simulink model "PubIfDecisionTOS_MDL"  (R2020b)
settings: configuration reference "DspaceConfig" (kept outside this file)
PostLoadFcn:
  | if any(exist('dsrtsu_mdlpostloadfcn', 'file') ~= 0), dsrtsu_mdlpostloadfcn('Execute', bdroot); end
InitFcn:
  | , if any(exist('dsmpb_private', 'file') ~= 0), dsmpb_private('dsmpb_mdlclblib', 'Init', bdroot); end,
undefined symbols (not defined in the file or in its folder): C_TOS_ACCEgoRAxletoFbumplength_m, C_TOS_ACCTargetFront_Flag, C_TOS_AEBJAPedObjDxThre_Val, C_TOS_AEBJAPedObjDyThre_Val, C_TOS_AEBJATargetSize_Val, C_TOS_AEBJAVehObjDxThre_Val, C_TOS_AEBJAVehObjDyThre_Val, C_TOS_AEBJuncPedTargetSize_Val, C_TOS_AEBLatObjDxThre_Val, C_TOS_AEBLatPedDyThre_Val, C_TOS_AEBLatTargetSize_Val, C_TOS_AEBLongTargetInEgoFront_Flag, C_TOS_axAbsGround_Parameter, C_TOS_CameraConfirmedFlag, C_TOS_CNsubjWidth, C_TOS_CurrentLaneCoreMinWidth_Val, C_TOS_CutInProb_Val_Zero, C_TOS_CutOutProb_Val_Zero, C_TOS_D2R_Val, C_TOS_DefaultValueObjectToCenterLine_dy, C_TOS_EgoCarWidth_Val, C_TOS_EgoDxRefPoint_m, C_TOS_EgoRAxletoFbumplength_m, C_TOS_HalfWidthVehicle_Con, C_TOS_HWA_CurrentLaneFlag, C_TOS_HWA_LeftLaneFlag, C_TOS_HWA_MovingDir_Vaild, C_TOS_HWA_MovState_Vaild, C_TOS_HWA_RightLaneFlag, C_TOS_LaneLineCourseErrorFront, C_TOS_LaneLineCourseErrorRear, C_TOS_MotorbikeDefaultWidth_m, C_TOS_NumberOfEffectiveTargets, C_TOS_Obj_Age_Val, C_TOS_Objdx_Constraint_Val, C_TOS_ObjectDefaultWidth_m, C_TOS_ObjInCurrentLane_Val, C_TOS_ObjInCurrentLaneValid, C_TOS_ObjInLeftLaneValid, C_TOS_ObjInRightLaneValid, C_TOS_ObjNotInCurrentLane_Val, C_TOS_ObjNotREElementType, C_TOS_ObjPredictDis_dy_ConstantVal_Zeros, C_TOS_ObjToCenterLine_ConstantVal_Zeros, C_TOS_OFMObjIDInvilad_Val, C_TOS_PIL_LatDisCons_Val_zero, C_TOS_PIL_ObjectCutInFlag_b, C_TOS_PIL_ObjectCutOutFlag_b, C_TOS_PIL_ObjLaneProb_al_Val, C_TOS_PP_ObjFusType_FC_Confirm_b, C_TOS_PP_ObjFusType_FC_FR_Confirm_b, C_TOS_PP_ObjFusType_FR_Confirm_b, C_TOS_RE_80BoolDefault_Val, C_TOS_RE_80Single181Default_Val, C_TOS_RE_80Single255Default_Val, C_TOS_RE_80Uint8Default_Val, C_TOS_RE_D2R, C_TOS_RE_D_180_Val, C_TOS_RE_InvalidObjectID_Val, C_TOS_RE_InvalidTargetChainDir_Val ... (+142)
libraries: simulink x1650, TOS_LIB x361, canfdmsglib x14
(part 27 of 69)

== system PubIfDecisionTOS_MDL/TOS_20201112/TOS_2012080320/TOS/ACC/TOS_ACCCurrentLane/ACC_CurrentLane_Target/TOS_ACC_P0/ACC_P0_Targe ==
  ACC_P0_Index : Inport
  Object_Fus_Type : Inport  Port=2
  object_MovingState : Inport  Port=3
  PP_ObjMovingDirSignalProcessing : Inport  Port=4
  Object_HeadingAngle : Inport  Port=5
  Object_DX : Inport  Port=6
  TOS_TLJ_SameLaneConfirm_Flag : Inport  Port=7
  Object_Type : Inport  Port=8
  Object_ObstacleProb : Inport  Port=9
  Object_DY : Inport  Port=10
  PP_ObjFusType_FC_FR_Confirm : Inport  Port=11
  PP_ObjFusType_FR_Confirm : Inport  Port=12
  PP_ObjFusType_FC_Confirm : Inport  Port=13
  Object_VX : Inport  Port=14
  Object_VY : Inport  Port=15
  VIE_EgoVelocity : Inport  Port=16
  SteerWheelAng : Inport  Port=17
  PIL_OverlapRatio : Inport  Port=18
  ACC_Target_ID_K1 : Inport  Port=19
  ACC_Target_ID_K2 : Inport  Port=20
  ACC_Target_MovState_K1 : Inport  Port=21
  ACC_Target_MovState_K2 : Inport  Port=22
  ObjectID : Inport  Port=23
  LM_LR_Line04_dDisStart : Inport  Port=24
  LM_LR_Line04_dDisEnd : Inport  Port=25
  LM_LR_Line05_dDisStart : Inport  Port=26
  LM_LR_Line05_dDisEnd : Inport  Port=27
  LM_LR_Line06_dDisStart : Inport  Port=28
  LM_LR_Line06_dDisEnd : Inport  Port=29
  LM_LR_Line04_pC2 : Inport  Port=30
  LM_LR_Line05_pC2 : Inport  Port=31
  LM_LR_Line06_pC2 : Inport  Port=32
  LM_LR_Line04_fCamValid : Inport  Port=33
  LM_LR_Line05_fCamValid : Inport  Port=34
  LM_LR_Line06_fCamValid : Inport  Port=35
  LM_LR_Line04_pC0 : Inport  Port=36
  LM_RL_Line04_pC0 : Inport  Port=37
  LM_LR_Line04_pC1 : Inport  Port=38
  LM_RL_Line04_pC1 : Inport  Port=39
  Action Port : ActionPort  ActionPortLabel=else
  ACC_P0_Targe : Subsystem
  Selector{1..16} (16 alike) : Selector  InputPortWidth=80  IndexOptions=Index vector (port)  Indices=[1 3]  OutputSizes=1
  ACC_P0_TargeConfirm : Outport
  TOS_ACC_FusionType_ObserVale : Outport  Port=2
  TOS_ACC_TrgMovDir_ObserVale : Outport  Port=3
  TOS_ACC_TargetDxConfirm_ObserVale : Outport  Port=4
  TOS_ACC_ObjType_ObserVale : Outport  Port=5
  TOS_ACC_ObstacleProb_ObserVale : Outport  Port=6
  TOS_ACC_DyConfirm_ObserVale : Outport  Port=7
  TOS_ACC_TrgMovDirFlag_1_ObserVale : Outport  Port=8
  TOS_ACC_TrgMovDirFlag_2_ObserVale : Outport  Port=9
  TOS_ACC_TrgMovDirFlag_3_ObserVale : Outport  Port=10
  TOS_ACC_TrgMovDirFlag_4_ObserVale : Outport  Port=11
  TOS_ACC_TrgMovDirFlag_5_ObserVale : Outport  Port=12
  TOS_ACC_TrgMovDirFlag_6_ObserVale : Outport  Port=13
  TOS_ACC_DyConfirm_1_ObserVale : Outport  Port=14
  TOS_ACC_DyConfirm_2_ObserVale : Outport  Port=15
  TOS_ACC_DyConfirm_3_ObserVale : Outport  Port=16
  TOS_ACC_DyConfirm_4_OverlapRatio_ObserVale : Outport  Port=17
  TOS_ACC_DyConfirm_5_OverlapConfirm_ObserVale : Outport  Port=18
  TOS_ACC_DyConfirm_ALL_6_ObserVale : Outport  Port=19
  wires:
  Object_Fus_Type/1 -> Selector1/1
  object_MovingState/1 -> Selector13/1
  PP_ObjMovingDirSignalProcessing/1 -> Selector12/1
  Object_HeadingAngle/1 -> Selector16/1
  Object_DX/1 -> Selector15/1
  TOS_TLJ_SameLaneConfirm_Flag/1 -> Selector14/1
  Object_Type/1 -> Selector11/1
  Object_ObstacleProb/1 -> Selector10/1
  Object_DY/1 -> Selector9/1
  PP_ObjFusType_FC_FR_Confirm/1 -> Selector8/1
  PP_ObjFusType_FR_Confirm/1 -> Selector7/1
  PP_ObjFusType_FC_Confirm/1 -> Selector6/1
  Object_VX/1 -> Selector5/1
  Object_VY/1 -> Selector2/1
  VIE_EgoVelocity/1 -> ACC_P0_Targe/15(VIE_EgoVelocity)
  SteerWheelAng/1 -> ACC_P0_Targe/16(SteerWheelAng)
  PIL_OverlapRatio/1 -> Selector4/1
  ACC_Target_ID_K1/1 -> ACC_P0_Targe/18(ACC_Target_ID_K1)
  ACC_Target_ID_K2/1 -> ACC_P0_Targe/19(ACC_Target_ID_K2)
  ACC_Target_MovState_K1/1 -> ACC_P0_Targe/20(ACC_Target_MovState_K1)
  ACC_Target_MovState_K2/1 -> ACC_P0_Targe/21(ACC_Target_MovState_K2)
  ObjectID/1 -> Selector3/1
  Selector1/1 -> ACC_P0_Targe/1(Object_Fus_Type)
  Selector13/1 -> ACC_P0_Targe/2(object_MovingState)
  Selector12/1 -> ACC_P0_Targe/3(PP_ObjMovingDirSignalProcessing)
  Selector16/1 -> ACC_P0_Targe/4(Object_HeadingAngle)
  Selector15/1 -> ACC_P0_Targe/5(Object_DX)
  Selector14/1 -> ACC_P0_Targe/6(TOS_TLJ_SameLaneConfirm_Flag)
  Selector11/1 -> ACC_P0_Targe/7(Object_Type)
  Selector10/1 -> ACC_P0_Targe/8(Object_ObstacleProb)
  Selector9/1 -> ACC_P0_Targe/9(Object_DY)
  Selector8/1 -> ACC_P0_Targe/10(PP_ObjFusType_FC_FR_Confirm)
  Selector7/1 -> ACC_P0_Targe/11(PP_ObjFusType_FR_Confirm)
  Selector6/1 -> ACC_P0_Targe/12(PP_ObjFusType_FC_Confirm)
  Selector5/1 -> ACC_P0_Targe/13(Object_VX)
  Selector2/1 -> ACC_P0_Targe/14(Object_VY)
  Selector4/1 -> ACC_P0_Targe/17(PIL_OverlapRatio)
  Selector3/1 -> ACC_P0_Targe/22(ObjectID)
  ACC_P0_Index/1 -> Selector1/2, Selector13/2, Selector12/2, Selector15/2, Selector3/2, Selector4/2, Selector2/2, Selector5/2, Selector6/2, Selector7/2, Selector8/2, Selector9/2, Selector10/2, Selector11/2, Selector14/2, Selector16/2
  LM_LR_Line06_pC2/1 -> ACC_P0_Targe/31(LM_LR_Line06_pC2)
  LM_LR_Line04_dDisStart/1 -> ACC_P0_Targe/23(LM_LR_Line04_dDisStart)
  LM_LR_Line04_dDisEnd/1 -> ACC_P0_Targe/24(LM_LR_Line04_dDisEnd)
  LM_LR_Line05_dDisStart/1 -> ACC_P0_Targe/25(LM_LR_Line05_dDisStart)
  LM_LR_Line05_dDisEnd/1 -> ACC_P0_Targe/26(LM_LR_Line05_dDisEnd)
  LM_LR_Line06_dDisStart/1 -> ACC_P0_Targe/27(LM_LR_Line06_dDisStart)
  LM_LR_Line06_dDisEnd/1 -> ACC_P0_Targe/28(LM_LR_Line06_dDisEnd)
  LM_LR_Line04_pC2/1 -> ACC_P0_Targe/29(LM_LR_Line04_pC2)
  LM_LR_Line05_pC2/1 -> ACC_P0_Targe/30(LM_LR_Line05_pC2)
  LM_LR_Line06_fCamValid/1 -> ACC_P0_Targe/34(LM_LR_Line06_fCamValid)
  LM_LR_Line04_fCamValid/1 -> ACC_P0_Targe/32(LM_LR_Line04_fCamValid)
  LM_LR_Line05_fCamValid/1 -> ACC_P0_Targe/33(LM_LR_Line05_fCamValid)
  ACC_P0_Targe/6(TOS_ACC_ObstacleProb_ObserVale) -> TOS_ACC_ObstacleProb_ObserVale/1
  ACC_P0_Targe/7(TOS_ACC_DyConfirm_ObserVale) -> TOS_ACC_DyConfirm_ObserVale/1
  ACC_P0_Targe/5(TOS_ACC_ObjType_ObserVale) -> TOS_ACC_ObjType_ObserVale/1
  ACC_P0_Targe/8(TOS_ACC_TrgMovDirFlag_1_ObserVale) -> TOS_ACC_TrgMovDirFlag_1_ObserVale/1
  ACC_P0_Targe/4(TOS_ACC_TargetDxConfirm_ObserVale) -> TOS_ACC_TargetDxConfirm_ObserVale/1
  ACC_P0_Targe/9(TOS_ACC_TrgMovDirFlag_2_ObserVale) -> TOS_ACC_TrgMovDirFlag_2_ObserVale/1
  ACC_P0_Targe/3(TOS_ACC_TrgMovDir_ObserVale) -> TOS_ACC_TrgMovDir_ObserVale/1
  ACC_P0_Targe/10(TOS_ACC_TrgMovDirFlag_3_ObserVale) -> TOS_ACC_TrgMovDirFlag_3_ObserVale/1
  ACC_P0_Targe/2(TOS_ACC_FusionType_ObserVale) -> TOS_ACC_FusionType_ObserVale/1
  ACC_P0_Targe/11(TOS_ACC_TrgMovDirFlag_4_ObserVale) -> TOS_ACC_TrgMovDirFlag_4_ObserVale/1
  ACC_P0_Targe/1(ACC_P0_TargeConfirm) -> ACC_P0_TargeConfirm/1
  ACC_P0_Targe/12(TOS_ACC_TrgMovDirFlag_5_ObserVale) -> TOS_ACC_TrgMovDirFlag_5_ObserVale/1
  ACC_P0_Targe/13(TOS_ACC_TrgMovDirFlag_6_ObserVale) -> TOS_ACC_TrgMovDirFlag_6_ObserVale/1
  ACC_P0_Targe/14(TOS_ACC_DyConfirm_1_ObserVale) -> TOS_ACC_DyConfirm_1_ObserVale/1
  ACC_P0_Targe/15(TOS_ACC_DyConfirm_2_ObserVale) -> TOS_ACC_DyConfirm_2_ObserVale/1
  ACC_P0_Targe/16(TOS_ACC_DyConfirm_3_ObserVale) -> TOS_ACC_DyConfirm_3_ObserVale/1
  ACC_P0_Targe/17(TOS_ACC_DyConfirm_4_OverlapRatio_ObserVale) -> TOS_ACC_DyConfirm_4_OverlapRatio_ObserVale/1
  ACC_P0_Targe/18(TOS_ACC_DyConfirm_5_OverlapConfirm_ObserVale) -> TOS_ACC_DyConfirm_5_OverlapConfirm_ObserVale/1
  ACC_P0_Targe/19(TOS_ACC_DyConfirm_ALL_6_ObserVale) -> TOS_ACC_DyConfirm_ALL_6_ObserVale/1
  LM_LR_Line04_pC0/1 -> ACC_P0_Targe/35(LM_LR_Line04_pC0)
  LM_RL_Line04_pC0/1 -> ACC_P0_Targe/36(LM_RL_Line04_pC0)
  LM_LR_Line04_pC1/1 -> ACC_P0_Targe/37(LM_LR_Line04_pC1)
  LM_RL_Line04_pC1/1 -> ACC_P0_Targe/38(LM_RL_Line04_pC1)

== system PubIfDecisionTOS_MDL/TOS_20201112/TOS_2012080320/TOS/ACC/TOS_ACCCurrentLane/ACC_CurrentLane_Target/TOS_ACC_P0/ACC_P0_TargeDefault ==
  Action Port : ActionPort  ActionPortLabel=if(u1 ~= 0)
  Constant{1..19} (19 alike) : Constant  Value=0  OutDataTypeStr=boolean
  ACC_P0_TargeConfirm : Outport
  TOS_ACC_FusionType_ObserVale : Outport  Port=2
  TOS_ACC_TrgMovDir_ObserVale : Outport  Port=3
  TOS_ACC_TargetDxConfirm_ObserVale : Outport  Port=4
  TOS_ACC_ObjType_ObserVale : Outport  Port=5
  TOS_ACC_ObstacleProb_ObserVale : Outport  Port=6
  TOS_ACC_DyConfirm_ObserVale : Outport  Port=7
  TOS_ACC_TrgMovDirFlag_1_ObserVale : Outport  Port=8
  TOS_ACC_TrgMovDirFlag_2_ObserVale : Outport  Port=9
  TOS_ACC_TrgMovDirFlag_3_ObserVale : Outport  Port=10
  TOS_ACC_TrgMovDirFlag_4_ObserVale : Outport  Port=11
  TOS_ACC_TrgMovDirFlag_5_ObserVale : Outport  Port=12
  TOS_ACC_TrgMovDirFlag_6_ObserVale : Outport  Port=13
  TOS_ACC_DyConfirm_1_ObserVale : Outport  Port=14
  TOS_ACC_DyConfirm_2_ObserVale : Outport  Port=15
  TOS_ACC_DyConfirm_3_ObserVale : Outport  Port=16
  TOS_ACC_DyConfirm_4_OverlapRatio_ObserVale : Outport  Port=17
  TOS_ACC_DyConfirm_5_OverlapConfirm_ObserVale : Outport  Port=18
  TOS_ACC_DyConfirm_ALL_6_ObserVale1 : Outport  Port=19
  wires:
  Constant2/1 -> ACC_P0_TargeConfirm/1
  Constant1/1 -> TOS_ACC_FusionType_ObserVale/1
  Constant3/1 -> TOS_ACC_TrgMovDir_ObserVale/1
  Constant4/1 -> TOS_ACC_TargetDxConfirm_ObserVale/1
  Constant5/1 -> TOS_ACC_ObjType_ObserVale/1
  Constant6/1 -> TOS_ACC_ObstacleProb_ObserVale/1
  Constant7/1 -> TOS_ACC_DyConfirm_ObserVale/1
  Constant8/1 -> TOS_ACC_TrgMovDirFlag_1_ObserVale/1
  Constant9/1 -> TOS_ACC_TrgMovDirFlag_2_ObserVale/1
  Constant10/1 -> TOS_ACC_TrgMovDirFlag_3_ObserVale/1
  Constant11/1 -> TOS_ACC_TrgMovDirFlag_4_ObserVale/1
  Constant12/1 -> TOS_ACC_TrgMovDirFlag_5_ObserVale/1
  Constant13/1 -> TOS_ACC_TrgMovDirFlag_6_ObserVale/1
  Constant14/1 -> TOS_ACC_DyConfirm_2_ObserVale/1
  Constant15/1 -> TOS_ACC_DyConfirm_3_ObserVale/1
  Constant16/1 -> TOS_ACC_DyConfirm_4_OverlapRatio_ObserVale/1
  Constant17/1 -> TOS_ACC_DyConfirm_1_ObserVale/1
  Constant18/1 -> TOS_ACC_DyConfirm_5_OverlapConfirm_ObserVale/1
  Constant19/1 -> TOS_ACC_DyConfirm_ALL_6_ObserVale1/1

== system PubIfDecisionTOS_MDL/TOS_20201112/TOS_2012080320/TOS/ACC/TOS_ACCCurrentLane/ACC_CurrentLane_Target/TOS_ACC_P1/ACC_P1_Targe ==
  ACC_P1_Index : Inport
  Object_Fus_Type : Inport  Port=2
  object_MovingState : Inport  Port=3
  PP_ObjMovingDirSignalProcessing : Inport  Port=4
  Object_HeadingAngle : Inport  Port=5
  Object_DX : Inport  Port=6
  TOS_TLJ_SameLaneConfirm_Flag : Inport  Port=7
  Object_Type : Inport  Port=8
  Object_ObstacleProb : Inport  Port=9
  Object_DY : Inport  Port=10
  PP_ObjFusType_FC_FR_Confirm : Inport  Port=11
  PP_ObjFusType_FR_Confirm : Inport  Port=12
  PP_ObjFusType_FC_Confirm : Inport  Port=13
  Object_VX : Inport  Port=14
  Object_VY : Inport  Port=15
  VIE_EgoVelocity : Inport  Port=16
  SteerWheelAng : Inport  Port=17
  PIL_OverlapRatio : Inport  Port=18
  ACC_Target_ID_K1 : Inport  Port=19
  ACC_Target_ID_K2 : Inport  Port=20
  ACC_Target_MovState_K1 : Inport  Port=21
  ACC_Target_MovState_K2 : Inport  Port=22
  ObjectID : Inport  Port=23
  LM_LR_Line04_dDisStart : Inport  Port=24
  LM_LR_Line04_dDisEnd : Inport  Port=25
  LM_LR_Line05_dDisStart : Inport  Port=26
  LM_LR_Line05_dDisEnd : Inport  Port=27
  LM_LR_Line06_dDisStart : Inport  Port=28
  LM_LR_Line06_dDisEnd : Inport  Port=29
  LM_LR_Line04_pC2 : Inport  Port=30
  LM_LR_Line05_pC2 : Inport  Port=31
  LM_LR_Line06_pC2 : Inport  Port=32
  LM_LR_Line04_fCamValid : Inport  Port=33
  LM_LR_Line05_fCamValid : Inport  Port=34
  LM_LR_Line06_fCamValid : Inport  Port=35
  LM_LR_Line04_pC0 : Inport  Port=36
  LM_RL_Line04_pC0 : Inport  Port=37
  Action Port : ActionPort  ActionPortLabel=else
  ACC_P1_Targe : Subsystem
  Selector{1..16} (16 alike) : Selector  InputPortWidth=80  IndexOptions=Index vector (port)  Indices=[1 3]  OutputSizes=1
  ACC_P1_TargeConfirm : Outport
  TOS_ACC_FusionType_ObserVale : Outport  Port=2
  TOS_ACC_TrgMovDir_ObserVale : Outport  Port=3
  TOS_ACC_TargetDxConfirm_ObserVale : Outport  Port=4
  TOS_ACC_ObjType_ObserVale : Outport  Port=5
  TOS_ACC_ObstacleProb_ObserVale : Outport  Port=6
  TOS_ACC_DyConfirm_ObserVale : Outport  Port=7
  TOS_ACC_TrgMovDirFlag_1_ObserVale : Outport  Port=8
  TOS_ACC_TrgMovDirFlag_2_ObserVale : Outport  Port=9
  TOS_ACC_TrgMovDirFlag_3_ObserVale : Outport  Port=10
  TOS_ACC_TrgMovDirFlag_4_ObserVale : Outport  Port=11
  TOS_ACC_TrgMovDirFlag_5_ObserVale : Outport  Port=12
  TOS_ACC_TrgMovDirFlag_6_ObserVale : Outport  Port=13
  TOS_ACC_DyConfirm_1_ObserVale : Outport  Port=14
  TOS_ACC_DyConfirm_2_ObserVale : Outport  Port=15
  TOS_ACC_DyConfirm_3_ObserVale : Outport  Port=16
  TOS_ACC_DyConfirm_4_OverlapRatio_ObserVale : Outport  Port=17
  TOS_ACC_DyConfirm_5_OverlapConfirm_ObserVale : Outport  Port=18
  TOS_ACC_DyConfirm_ALL_6_ObserVale : Outport  Port=19
  wires:
  LM_RL_Line04_pC0/1 -> ACC_P1_Targe/36(LM_RL_Line04_pC0)
  LM_LR_Line04_pC0/1 -> ACC_P1_Targe/35(LM_LR_Line04_pC0)
  ACC_P1_Targe/19(TOS_ACC_DyConfirm_ALL_6_ObserVale) -> TOS_ACC_DyConfirm_ALL_6_ObserVale/1
  ACC_P1_Targe/18(TOS_ACC_DyConfirm_5_OverlapConfirm_ObserVale) -> TOS_ACC_DyConfirm_5_OverlapConfirm_ObserVale/1
  ACC_P1_Targe/17(TOS_ACC_DyConfirm_4_OverlapRatio_ObserVale) -> TOS_ACC_DyConfirm_4_OverlapRatio_ObserVale/1
  ACC_P1_Targe/16(TOS_ACC_DyConfirm_3_ObserVale) -> TOS_ACC_DyConfirm_3_ObserVale/1
  ACC_P1_Targe/15(TOS_ACC_DyConfirm_2_ObserVale) -> TOS_ACC_DyConfirm_2_ObserVale/1
  ACC_P1_Targe/14(TOS_ACC_DyConfirm_1_ObserVale) -> TOS_ACC_DyConfirm_1_ObserVale/1
  ACC_P1_Targe/13(TOS_ACC_TrgMovDirFlag_6_ObserVale) -> TOS_ACC_TrgMovDirFlag_6_ObserVale/1
  ACC_P1_Targe/12(TOS_ACC_TrgMovDirFlag_5_ObserVale) -> TOS_ACC_TrgMovDirFlag_5_ObserVale/1
  ACC_P1_Targe/1(ACC_P1_TargeConfirm) -> ACC_P1_TargeConfirm/1
  ACC_P1_Targe/11(TOS_ACC_TrgMovDirFlag_4_ObserVale) -> TOS_ACC_TrgMovDirFlag_4_ObserVale/1
  ACC_P1_Targe/2(TOS_ACC_FusionType_ObserVale) -> TOS_ACC_FusionType_ObserVale/1
  ACC_P1_Targe/10(TOS_ACC_TrgMovDirFlag_3_ObserVale) -> TOS_ACC_TrgMovDirFlag_3_ObserVale/1
  ACC_P1_Targe/3(TOS_ACC_TrgMovDir_ObserVale) -> TOS_ACC_TrgMovDir_ObserVale/1
  ACC_P1_Targe/9(TOS_ACC_TrgMovDirFlag_2_ObserVale) -> TOS_ACC_TrgMovDirFlag_2_ObserVale/1
  ACC_P1_Targe/4(TOS_ACC_TargetDxConfirm_ObserVale) -> TOS_ACC_TargetDxConfirm_ObserVale/1
  ACC_P1_Targe/8(TOS_ACC_TrgMovDirFlag_1_ObserVale) -> TOS_ACC_TrgMovDirFlag_1_ObserVale/1
  ACC_P1_Targe/5(TOS_ACC_ObjType_ObserVale) -> TOS_ACC_ObjType_ObserVale/1
  ACC_P1_Targe/7(TOS_ACC_DyConfirm_ObserVale) -> TOS_ACC_DyConfirm_ObserVale/1
  ACC_P1_Targe/6(TOS_ACC_ObstacleProb_ObserVale) -> TOS_ACC_ObstacleProb_ObserVale/1
  LM_LR_Line05_fCamValid/1 -> ACC_P1_Targe/33(LM_LR_Line05_fCamValid)
  LM_LR_Line04_fCamValid/1 -> ACC_P1_Targe/32(LM_LR_Line04_fCamValid)
  LM_LR_Line06_fCamValid/1 -> ACC_P1_Targe/34(LM_LR_Line06_fCamValid)
  LM_LR_Line05_pC2/1 -> ACC_P1_Targe/30(LM_LR_Line05_pC2)
  LM_LR_Line04_pC2/1 -> ACC_P1_Targe/29(LM_LR_Line04_pC2)
  LM_LR_Line06_dDisEnd/1 -> ACC_P1_Targe/28(LM_LR_Line06_dDisEnd)
  LM_LR_Line06_dDisStart/1 -> ACC_P1_Targe/27(LM_LR_Line06_dDisStart)
  LM_LR_Line05_dDisEnd/1 -> ACC_P1_Targe/26(LM_LR_Line05_dDisEnd)
  LM_LR_Line05_dDisStart/1 -> ACC_P1_Targe/25(LM_LR_Line05_dDisStart)
  LM_LR_Line04_dDisEnd/1 -> ACC_P1_Targe/24(LM_LR_Line04_dDisEnd)
  LM_LR_Line04_dDisStart/1 -> ACC_P1_Targe/23(LM_LR_Line04_dDisStart)
  LM_LR_Line06_pC2/1 -> ACC_P1_Targe/31(LM_LR_Line06_pC2)
  ACC_P1_Index/1 -> Selector16/2, Selector14/2, Selector11/2, Selector10/2, Selector9/2, Selector8/2, Selector7/2, Selector6/2, Selector5/2, Selector2/2, Selector4/2, Selector3/2, Selector15/2, Selector12/2, Selector13/2, Selector1/2
  Selector3/1 -> ACC_P1_Targe/22(ObjectID)
  Selector4/1 -> ACC_P1_Targe/17(PIL_OverlapRatio)
  Selector2/1 -> ACC_P1_Targe/14(Object_VY)
  Selector5/1 -> ACC_P1_Targe/13(Object_VX)
  Selector6/1 -> ACC_P1_Targe/12(PP_ObjFusType_FC_Confirm)
  Selector7/1 -> ACC_P1_Targe/11(PP_ObjFusType_FR_Confirm)
  Selector8/1 -> ACC_P1_Targe/10(PP_ObjFusType_FC_FR_Confirm)
  Selector9/1 -> ACC_P1_Targe/9(Object_DY)
  Selector10/1 -> ACC_P1_Targe/8(Object_ObstacleProb)
  Selector11/1 -> ACC_P1_Targe/7(Object_Type)
  Selector14/1 -> ACC_P1_Targe/6(TOS_TLJ_SameLaneConfirm_Flag)
  Selector15/1 -> ACC_P1_Targe/5(Object_DX)
  Selector16/1 -> ACC_P1_Targe/4(Object_HeadingAngle)
  Selector12/1 -> ACC_P1_Targe/3(PP_ObjMovingDirSignalProcessing)
  Selector13/1 -> ACC_P1_Targe/2(object_MovingState)
  Selector1/1 -> ACC_P1_Targe/1(Object_Fus_Type)
  ObjectID/1 -> Selector3/1
  ACC_Target_MovState_K2/1 -> ACC_P1_Targe/21(ACC_Target_MovState_K2)
  ACC_Target_MovState_K1/1 -> ACC_P1_Targe/20(ACC_Target_MovState_K1)
  ACC_Target_ID_K2/1 -> ACC_P1_Targe/19(ACC_Target_ID_K2)
  ACC_Target_ID_K1/1 -> ACC_P1_Targe/18(ACC_Target_ID_K1)
  PIL_OverlapRatio/1 -> Selector4/1
  SteerWheelAng/1 -> ACC_P1_Targe/16(SteerWheelAng)
  VIE_EgoVelocity/1 -> ACC_P1_Targe/15(VIE_EgoVelocity)
  Object_VY/1 -> Selector2/1
  Object_VX/1 -> Selector5/1
  PP_ObjFusType_FC_Confirm/1 -> Selector6/1
  PP_ObjFusType_FR_Confirm/1 -> Selector7/1
  PP_ObjFusType_FC_FR_Confirm/1 -> Selector8/1
  Object_DY/1 -> Selector9/1
  Object_ObstacleProb/1 -> Selector10/1
  Object_Type/1 -> Selector11/1
  TOS_TLJ_SameLaneConfirm_Flag/1 -> Selector14/1
  Object_DX/1 -> Selector15/1
  Object_HeadingAngle/1 -> Selector16/1
  PP_ObjMovingDirSignalProcessing/1 -> Selector12/1
  object_MovingState/1 -> Selector13/1
  Object_Fus_Type/1 -> Selector1/1

== system PubIfDecisionTOS_MDL/TOS_20201112/TOS_2012080320/TOS/ACC/TOS_ACCCurrentLane/ACC_CurrentLane_Target/TOS_ACC_P1/ACC_P1_TargeDefault ==
  Action Port : ActionPort  ActionPortLabel=if(u1 ~= 0)
  Constant{1..19} (19 alike) : Constant  Value=0  OutDataTypeStr=boolean
  ACC_P1_TargeConfirm : Outport
  TOS_ACC_FusionType_ObserVale : Outport  Port=2
  TOS_ACC_TrgMovDir_ObserVale : Outport  Port=3
  TOS_ACC_TargetDxConfirm_ObserVale : Outport  Port=4
  TOS_ACC_ObjType_ObserVale : Outport  Port=5
  TOS_ACC_ObstacleProb_ObserVale : Outport  Port=6
  TOS_ACC_DyConfirm_ObserVale : Outport  Port=7
  TOS_ACC_TrgMovDirFlag_1_ObserVale : Outport  Port=8
  TOS_ACC_TrgMovDirFlag_2_ObserVale : Outport  Port=9
  TOS_ACC_TrgMovDirFlag_3_ObserVale : Outport  Port=10
  TOS_ACC_TrgMovDirFlag_4_ObserVale : Outport  Port=11
  TOS_ACC_TrgMovDirFlag_5_ObserVale : Outport  Port=12
  TOS_ACC_TrgMovDirFlag_6_ObserVale : Outport  Port=13
  TOS_ACC_DyConfirm_1_ObserVale : Outport  Port=14
  TOS_ACC_DyConfirm_2_ObserVale : Outport  Port=15
  TOS_ACC_DyConfirm_3_ObserVale : Outport  Port=16
  TOS_ACC_DyConfirm_4_OverlapRatio_ObserVale : Outport  Port=17
  TOS_ACC_DyConfirm_5_OverlapConfirm_ObserVale : Outport  Port=18
  TOS_ACC_DyConfirm_ALL_6_ObserVale1 : Outport  Port=19
  wires:
  Constant19/1 -> TOS_ACC_DyConfirm_ALL_6_ObserVale1/1
  Constant18/1 -> TOS_ACC_DyConfirm_5_OverlapConfirm_ObserVale/1
  Constant17/1 -> TOS_ACC_DyConfirm_1_ObserVale/1
  Constant16/1 -> TOS_ACC_DyConfirm_4_OverlapRatio_ObserVale/1
  Constant15/1 -> TOS_ACC_DyConfirm_3_ObserVale/1
  Constant14/1 -> TOS_ACC_DyConfirm_2_ObserVale/1
  Constant13/1 -> TOS_ACC_TrgMovDirFlag_6_ObserVale/1
  Constant12/1 -> TOS_ACC_TrgMovDirFlag_5_ObserVale/1
  Constant11/1 -> TOS_ACC_TrgMovDirFlag_4_ObserVale/1
  Constant10/1 -> TOS_ACC_TrgMovDirFlag_3_ObserVale/1
  Constant9/1 -> TOS_ACC_TrgMovDirFlag_2_ObserVale/1
  Constant8/1 -> TOS_ACC_TrgMovDirFlag_1_ObserVale/1
  Constant7/1 -> TOS_ACC_DyConfirm_ObserVale/1
  Constant6/1 -> TOS_ACC_ObstacleProb_ObserVale/1
  Constant5/1 -> TOS_ACC_ObjType_ObserVale/1
  Constant4/1 -> TOS_ACC_TargetDxConfirm_ObserVale/1
  Constant3/1 -> TOS_ACC_TrgMovDir_ObserVale/1
  Constant1/1 -> TOS_ACC_FusionType_ObserVale/1
  Constant2/1 -> ACC_P1_TargeConfirm/1

== system PubIfDecisionTOS_MDL/TOS_20201112/TOS_2012080320/TOS/ACC/TOS_ACCCurrentLane/ACC_Object_PreConfirm/ACC_P0_P1_Object_TargPreConfirm/ACC_P0_P1_Object_TargPreConfirm ==
  note: 行人、自行车目标过滤
  note: 判断是否为护栏目标
  note: 针对，选中目标后，过滤突然出现的纵向距离更近的单雷达静止目标
  Object_ID : Inport
  PP_ObjFusType_FC_FR_Confirm : Inport  Port=2
  PP_ObjFusType_FR_Confirm : Inport  Port=3
  PP_ObjFusType_FC_Confirm : Inport  Port=4
  Obj_MovingState : Inport  Port=5
  Obj_Dx : Inport  Port=6
  Object_ObstacleProb : Inport  Port=7
  Object_DY : Inport  Port=8
  Object_ObjType : Inport  Port=9
  TOS_TLJ_SameLaneConfirm_Flag : Inport  Port=10
  LM_LR_Line04_fCamValid : Inport  Port=11
  LM_LR_Line05_fCamValid : Inport  Port=12
  LM_LR_Line06_fCamValid : Inport  Port=13
  ACC_TargetP0_ID_K1 : Inport  Port=14
  ACC_TargetP0_Dx_K1 : Inport  Port=15
  PIL_OverlapRatio : Inport  Port=16
  PIL_OverlapRatio_K1 : Inport  Port=17
  PIL_OverlapRatio_K2 : Inport  Port=18
  LM_LR_Line04_dDisStart : Inport  Port=19
  LM_LR_Line04_dDisEnd : Inport  Port=20
  LM_LR_Line05_dDisStart : Inport  Port=21
  LM_LR_Line05_dDisEnd : Inport  Port=22
  LM_LR_Line06_dDisStart : Inport  Port=23
  LM_LR_Line06_dDisEnd : Inport  Port=24
  PP_REElementType : Inport  Port=25
  Action Port : ActionPort  ActionPortLabel=else
  " " : Subsystem
  Bus Creator : BusCreator  Inputs=25
  Bus Selector1 : BusSelector  OutputSignals=PP_ObjFusType_FR_Confirm,Obj_MovingState,Obj_Dx,ACC_TargetP0_ID_K1,ACC_TargetP0_Dx_K1,Object_ID
  Bus Selector2 : BusSelector  OutputSignals=PP_ObjFusType_FC_FR_Confirm,PP_ObjFusType_FC_Confirm,PP_ObjFusType_FR_Confirm
  Bus Selector3 : BusSelector  OutputSignals=PP_ObjFusType_FR_Confirm,Obj_MovingState,Object_ObstacleProb,Object_DY
  Bus Selector4 : BusSelector  OutputSignals=Obj_MovingState,Object_ObjType
  Bus Selector5 : BusSelector  OutputSignals=PIL_OverlapRatio
  Bus Selector6 : BusSelector  OutputSignals=TOS_TLJ_SameLaneConfirm_Flag
  Bus Selector7 : BusSelector  OutputSignals=PP_REElementType
  Compare To Constant : simulink/Logic and Bit Operations/Compare To Constant  relop=>=  const=P_TOS_ACC_P0_P1_TargetPre_OverlapThre_Val  OutDataTypeStr=boolean
      settings: AttributesFormatString=P_TOS_ACC_P0_P1_TargetPre_OverlapThre_Val = 0.05
  Compare To Constant2 : simulink/Logic and Bit Operations/Compare To Constant  relop===  const=C_TOS_ACCTargetFront_Flag  OutDataTypeStr=boolean
      settings: AttributesFormatString=C_TOS_ACCTargetFront_Flag = 1
  Constant : Constant  Value=0  OutDataTypeStr=single
  Logical Operator : Logic  Operator=NOT  AllPortsSameDT=off  OutDataTypeStr=boolean
  Logical Operator1 : Logic  Inputs=6  AllPortsSameDT=off  OutDataTypeStr=boolean
  Logical Operator2 : Logic  Operator=NOT  AllPortsSameDT=off  OutDataTypeStr=boolean
  Logical Operator3 : Logic  Operator=OR  AllPortsSameDT=off  OutDataTypeStr=boolean
  Overlap : Subsystem
  Subsystem : Subsystem
  Subsystem1 : Subsystem
  Subsystem2 : Subsystem
  Subsystem3 : Subsystem
  Switch : Switch  Criteria=u2 > Threshold
  TOS_ACC_DyConfirm : Subsystem
  TOS_ACC_P0_P1_TargetPre_1_ConditionFlag_ObserVale : Outport
  TOS_ACC_P0_P1_TargetPre_2_OverlapThre_ObserVale : Outport  Port=2
  TOS_ACC_P0_P1_TargetPre_3_SameLane_Flag_ObserVale : Outport  Port=3
  TOS_ACC_P0_P1_TargetPre_SameLaneFlag : Outport  Port=4
  TOS_ACC_P0_P1_TargetPre_FiltFlag : Outport  Port=5
  TOS_ACC_P0_P1_TargetPre_FusionTypeFlag_ObserVale : Outport  Port=6
  TOS_ACC_P0_P1_TargetPre_PassedbyTarget_Flag_ObserVale : Outport  Port=7
  TOS_ACC_P0_P1_TargetPre_FenceFlag_ObserVale : Outport  Port=8
  TOS_ACC_P0_P1_TargetPre_ObjType_ObserVale : Outport  Port=9
  TOS_ACC_P0_P1_TargetPre_OverlapThre_Val_ObserVale : Outport  Port=10
  TOS_ACC_P0_P1_TargetPre_REElementType_ObserVale : Outport  Port=11
  wires:
  Subsystem/1(TOS_ACC_P0_P1_TargetPre_TargetFusionTypeFlag) -> [TOS_ACC_P0_P1_TargetPre_FusionTypeFlag_ObserVale], Logical Operator1/1
  Subsystem1/1(TOS_ACC_P0_P1_TargetPre_ObjectPassedbyTarget_Flag) -> Logical Operator/1
  Subsystem3/1(TOS_ACC_P0_P1_TargetPre_FenceFlag) -> Logical Operator2/1
  Logical Operator2/1 -> [TOS_ACC_P0_P1_TargetPre_FenceFlag_ObserVale], Logical Operator1/3
  Logical Operator/1 -> [TOS_ACC_P0_P1_TargetPre_PassedbyTarget_Flag_ObserVale], Logical Operator1/2
  Bus Selector1/6 -> Subsystem1/6(Object_ID)  "<Object_ID>"
  PP_ObjFusType_FR_Confirm/1 -> Bus Creator/3  "PP_ObjFusType_FR_Confirm"
  Bus Selector1/4 -> Subsystem1/4(ACC_TargetP0_ID_K1)  "<ACC_TargetP0_ID_K1>"
  Object_ID/1 -> Bus Creator/1  "Object_ID"
  PP_ObjFusType_FC_Confirm/1 -> Bus Creator/4  "PP_ObjFusType_FC_Confirm"
  Bus Selector2/1 -> Subsystem/1(PP_ObjFusType_FC_FR_Confirm)  "<PP_ObjFusType_FC_FR_Confirm>"
  Bus Selector2/3 -> Subsystem/3(PP_ObjFusType_FC_Confirm)  "<PP_ObjFusType_FR_Confirm>"
  Bus Selector1/1 -> Subsystem1/1(FR_Confirm)  "<PP_ObjFusType_FR_Confirm>"
  Bus Selector2/2 -> Subsystem/2(PP_ObjFusType_FR_Confirm)  "<PP_ObjFusType_FC_Confirm>"
  Bus Selector1/5 -> Subsystem1/5(ACC_TargetP0_Dx_K1)  "<ACC_TargetP0_Dx_K1>"
  PP_ObjFusType_FC_FR_Confirm/1 -> Bus Creator/2  "PP_ObjFusType_FC_FR_Confirm"
  ACC_TargetP0_ID_K1/1 -> Bus Creator/14  "ACC_TargetP0_ID_K1"
  Object_DY/1 -> Bus Creator/8  "Object_DY"
  Bus Selector1/2 -> Subsystem1/2(Obj_MovingState)  "<Obj_MovingState>"
  Bus Selector3/2 -> Subsystem3/2(Obj_MovingState)  "<Obj_MovingState>"
  ACC_TargetP0_Dx_K1/1 -> Bus Creator/15  "ACC_TargetP0_Dx_K1"
  Obj_MovingState/1 -> Bus Creator/5  "Obj_MovingState"
  Bus Selector1/3 -> Subsystem1/3(Obj_Dx)  "<Obj_Dx>"
  Object_ObstacleProb/1 -> Bus Creator/7  "Object_ObstacleProb"
  Bus Selector3/3 -> Subsystem3/3(Object_ObstacleProb)  "<Object_ObstacleProb>"
  Bus Selector3/4 -> Subsystem3/4(Object_DY)  "<Object_DY>"
  Bus Selector3/1 -> Subsystem3/1(FR_Confirm)  "<PP_ObjFusType_FR_Confirm>"
  Obj_Dx/1 -> Bus Creator/6  "Obj_Dx"
  Bus Selector4/2 -> " "/2(Object_Type)  "<Object_ObjType>"
  Bus Selector4/1 -> " "/1(object_MovingState)  "<Obj_MovingState>"
  " "/1(TOS_ACC_P0_P1_ObjType) -> [TOS_ACC_P0_P1_TargetPre_ObjType_ObserVale], Logical Operator1/4
  Object_ObjType/1 -> Bus Creator/9  "Object_ObjType"
  [TOS_ACC_P0_P1_TargetPre_FusionTypeFlag_ObserVale] -> TOS_ACC_P0_P1_TargetPre_FusionTypeFlag_ObserVale/1
  [TOS_ACC_P0_P1_TargetPre_PassedbyTarget_Flag_ObserVale] -> TOS_ACC_P0_P1_TargetPre_PassedbyTarget_Flag_ObserVale/1
  [TOS_ACC_P0_P1_TargetPre_FenceFlag_ObserVale] -> TOS_ACC_P0_P1_TargetPre_FenceFlag_ObserVale/1
  [TOS_ACC_P0_P1_TargetPre_ObjType_ObserVale] -> TOS_ACC_P0_P1_TargetPre_ObjType_ObserVale/1
  PIL_OverlapRatio/1 -> Bus Creator/16  "PIL_OverlapRatio"
  Bus Selector5/1 -> Compare To Constant/1  "<PIL_OverlapRatio>"
  Switch/1 -> [TOS_ACC_P0_P1_TargetPre_OverlapThre_Val_ObserVale], Logical Operator1/5
  [TOS_ACC_P0_P1_TargetPre_OverlapThre_Val_ObserVale] -> TOS_ACC_P0_P1_TargetPre_OverlapThre_Val_ObserVale/1
  TOS_TLJ_SameLaneConfirm_Flag/1 -> Bus Creator/10  "TOS_TLJ_SameLaneConfirm_Flag"
  Bus Selector6/1 -> Compare To Constant2/1  "<TOS_TLJ_SameLaneConfirm_Flag>"
  Compare To Constant2/1 -> [TOS_ACC_P0_P1_TargetPre_3_SameLane_Flag_ObserVale], Logical Operator3/2
  Logical Operator3/1 -> TOS_ACC_P0_P1_TargetPre_SameLaneFlag/1
  Logical Operator1/1 -> [TOS_ACC_P0_P1_TargetPre_1_ConditionFlag_ObserVale], TOS_ACC_P0_P1_TargetPre_FiltFlag/1
  [TOS_ACC_P0_P1_TargetPre_2_OverlapThre_ObserVale] -> TOS_ACC_P0_P1_TargetPre_2_OverlapThre_ObserVale/1
  [TOS_ACC_P0_P1_TargetPre_3_SameLane_Flag_ObserVale] -> TOS_ACC_P0_P1_TargetPre_3_SameLane_Flag_ObserVale/1
  [TOS_ACC_P0_P1_TargetPre_1_ConditionFlag_ObserVale] -> TOS_ACC_P0_P1_TargetPre_1_ConditionFlag_ObserVale/1
  PIL_OverlapRatio_K1/1 -> Bus Creator/17  "PIL_OverlapRatio_K1"
  PIL_OverlapRatio_K2/1 -> Bus Creator/18  "PIL_OverlapRatio_K2"
  LM_LR_Line04_fCamValid/1 -> Bus Creator/11  "LM_LR_Line04_fCamValid"
  LM_LR_Line05_fCamValid/1 -> Bus Creator/12  "LM_LR_Line05_fCamValid"
  LM_LR_Line06_fCamValid/1 -> Bus Creator/13  "LM_LR_Line06_fCamValid"
  LM_LR_Line04_dDisStart/1 -> Bus Creator/19  "LM_LR_Line04_dDisStart"
  LM_LR_Line04_dDisEnd/1 -> Bus Creator/20  "LM_LR_Line04_dDisEnd"
  LM_LR_Line05_dDisStart/1 -> Bus Creator/21  "LM_LR_Line05_dDisStart"
  LM_LR_Line05_dDisEnd/1 -> Bus Creator/22  "LM_LR_Line05_dDisEnd"
  LM_LR_Line06_dDisStart/1 -> Bus Creator/23  "LM_LR_Line06_dDisStart"
  LM_LR_Line06_dDisEnd/1 -> Bus Creator/24  "LM_LR_Line06_dDisEnd"
  Overlap/1(Overlap) -> [TOS_ACC_P0_P1_TargetPre_2_OverlapThre_ObserVale], Logical Operator3/1
  TOS_ACC_DyConfirm/1(TOS_ACC_DyConfirm) -> Switch/3
  Compare To Constant/1 -> Switch/1
  Constant/1 -> Switch/2
  Bus Selector7/1 -> Subsystem2/1(<PP_REElementType>)  "<PP_REElementType>"
  Subsystem2/1(TOS_ACC_P0_P1_REElementType) -> Logical Operator1/6, [TOS_ACC_P0_P1_REElementType_ObserVale]
  Bus Creator/1 -> Bus Selector6/1, Overlap/1(LM), Bus Selector7/1, TOS_ACC_DyConfirm/1(TOS_ACC_P0_P1_Dy), Bus Selector5/1, Bus Selector4/1, Bus Selector3/1, Bus Selector1/1, Bus Selector2/1
  [TOS_ACC_P0_P1_REElementType_ObserVale] -> TOS_ACC_P0_P1_TargetPre_REElementType_ObserVale/1
  PP_REElementType/1 -> Bus Creator/25  "PP_REElementType"

== system PubIfDecisionTOS_MDL/TOS_20201112/TOS_2012080320/TOS/ACC/TOS_ACCCurrentLane/ACC_Object_PreConfirm/ACC_P0_P1_Object_TargPreConfirm/ACC_P0_P1_Object_TargPreConfirmDefault ==
  Action Port : ActionPort  ActionPortLabel=if(u1 ~= 0)
  Constant{1..11} (11 alike) : Constant  Value=0  OutDataTypeStr=boolean
  TOS_ACC_P0_P1_TargetPre_1_ConditionFlag_ObserVale : Outport
  TOS_ACC_P0_P1_TargetPre_2_OverlapThre_ObserVale : Outport  Port=2
  TOS_ACC_P0_P1_TargetPre_3_SameLane_Flag_ObserVale : Outport  Port=3
  TOS_ACC_P0_P1_TargetPre_SameLaneFlag : Outport  Port=4
  TOS_ACC_P0_P1_TargetPre_FiltFlag : Outport  Port=5
  TOS_ACC_P0_P1_TargetPre_FusionTypeFlag_ObserVale : Outport  Port=6
  TOS_ACC_P0_P1_TargetPre_PassedbyTarget_Flag_ObserVale : Outport  Port=7
  TOS_ACC_P0_P1_TargetPre_FenceFlag_ObserVale : Outport  Port=8
  TOS_ACC_P0_P1_TargetPre_ObjType_ObserVale : Outport  Port=9
  TOS_ACC_P0_P1_TargetPre_OverlapThre_Val_ObserVale : Outport  Port=10
  TOS_ACC_P0_P1_TargetPre_REElementType_ObserVale : Outport  Port=11
  wires:
  Constant2/1 -> TOS_ACC_P0_P1_TargetPre_1_ConditionFlag_ObserVale/1
  Constant9/1 -> TOS_ACC_P0_P1_TargetPre_OverlapThre_Val_ObserVale/1
  Constant1/1 -> TOS_ACC_P0_P1_TargetPre_2_OverlapThre_ObserVale/1
  Constant3/1 -> TOS_ACC_P0_P1_TargetPre_3_SameLane_Flag_ObserVale/1
  Constant4/1 -> TOS_ACC_P0_P1_TargetPre_SameLaneFlag/1
  Constant5/1 -> TOS_ACC_P0_P1_TargetPre_FiltFlag/1
  Constant6/1 -> TOS_ACC_P0_P1_TargetPre_FusionTypeFlag_ObserVale/1
  Constant7/1 -> TOS_ACC_P0_P1_TargetPre_PassedbyTarget_Flag_ObserVale/1
  Constant8/1 -> TOS_ACC_P0_P1_TargetPre_FenceFlag_ObserVale/1
  Constant10/1 -> TOS_ACC_P0_P1_TargetPre_ObjType_ObserVale/1
  Constant11/1 -> TOS_ACC_P0_P1_TargetPre_REElementType_ObserVale/1

== system PubIfDecisionTOS_MDL/TOS_20201112/TOS_2012080320/TOS/ACC/TOS_ACCLeftLane/ACC_LeftLane_Target/TOS_ACC_P2/ACC_P2_Targe ==
  ACC_P2_Index : Inport
  Object_Fus_Type : Inport  Port=2
  object_MovingState : Inport  Port=3
  PP_ObjMovingDirSignalProcessing : Inport  Port=4
  Object_HeadingAngle : Inport  Port=5
  Object_DX : Inport  Port=6
  Object_Type : Inport  Port=7
  Object_ObstacleProb : Inport  Port=8
  Object_DY : Inport  Port=9
  PP_ObjFusType_FC_FR_Confirm : Inport  Port=10
  PP_ObjFusType_FR_Confirm : Inport  Port=11
  PP_ObjFusType_FC_Confirm : Inport  Port=12
  Object_VX : Inport  Port=13
  Object_VY : Inport  Port=14
  VIE_EgoVelocity : Inport  Port=15
  SteerWheelAng : Inport  Port=16
  ACC_Target_ID_K1 : Inport  Port=17
  ACC_Target_ID_K2 : Inport  Port=18
  ACC_Target_MovState_K1 : Inport  Port=19
  ACC_Target_MovState_K2 : Inport  Port=20
  ObjectID : Inport  Port=21
  Action Port : ActionPort  ActionPortLabel=else
  ACC_P2_Targe : Subsystem
  Selector{1..3,5..13,15..16} (14 alike) : Selector  InputPortWidth=80  IndexOptions=Index vector (port)  Indices=[1 3]  OutputSizes=1
  ACC_P2_TargeConfirm : Outport
  TOS_ACC_FusionType_ObserVale : Outport  Port=2
  TOS_ACC_TrgMovDir_ObserVale : Outport  Port=3
  TOS_ACC_TargetDxConfirm_ObserVale : Outport  Port=4
  TOS_ACC_ObjType_ObserVale : Outport  Port=5
  TOS_ACC_ObstacleProb_ObserVale : Outport  Port=6
  TOS_ACC_TrgMovDirFlag_1_ObserVale : Outport  Port=7
  TOS_ACC_TrgMovDirFlag_2_ObserVale : Outport  Port=8
  TOS_ACC_TrgMovDirFlag_3_ObserVale : Outport  Port=9
  TOS_ACC_TrgMovDirFlag_4_ObserVale : Outport  Port=10
  TOS_ACC_TrgMovDirFlag_5_ObserVale : Outport  Port=11
  TOS_ACC_TrgMovDirFlag_6_ObserVale : Outport  Port=12
  wires:
  ACC_P2_Targe/12(TOS_ACC_TrgMovDirFlag_6_ObserVale) -> TOS_ACC_TrgMovDirFlag_6_ObserVale/1
  ACC_P2_Targe/11(TOS_ACC_TrgMovDirFlag_5_ObserVale) -> TOS_ACC_TrgMovDirFlag_5_ObserVale/1
  ACC_P2_Targe/1(ACC_P2_TargeConfirm) -> ACC_P2_TargeConfirm/1
  ACC_P2_Targe/10(TOS_ACC_TrgMovDirFlag_4_ObserVale) -> TOS_ACC_TrgMovDirFlag_4_ObserVale/1
  ACC_P2_Targe/2(TOS_ACC_FusionType_ObserVale) -> TOS_ACC_FusionType_ObserVale/1
  ACC_P2_Targe/9(TOS_ACC_TrgMovDirFlag_3_ObserVale) -> TOS_ACC_TrgMovDirFlag_3_ObserVale/1
  ACC_P2_Targe/3(TOS_ACC_TrgMovDir_ObserVale) -> TOS_ACC_TrgMovDir_ObserVale/1
  ACC_P2_Targe/8(TOS_ACC_TrgMovDirFlag_2_ObserVale) -> TOS_ACC_TrgMovDirFlag_2_ObserVale/1
  ACC_P2_Targe/4(TOS_ACC_TargetDxConfirm_ObserVale) -> TOS_ACC_TargetDxConfirm_ObserVale/1
  ACC_P2_Targe/7(TOS_ACC_TrgMovDirFlag_1_ObserVale) -> TOS_ACC_TrgMovDirFlag_1_ObserVale/1
  ACC_P2_Targe/5(TOS_ACC_ObjType_ObserVale) -> TOS_ACC_ObjType_ObserVale/1
  ACC_P2_Targe/6(TOS_ACC_ObstacleProb_ObserVale) -> TOS_ACC_ObstacleProb_ObserVale/1
  ACC_P2_Index/1 -> Selector16/2, Selector3/2, Selector2/2, Selector5/2, Selector6/2, Selector7/2, Selector8/2, Selector9/2, Selector10/2, Selector11/2, Selector15/2, Selector12/2, Selector13/2, Selector1/2
  Selector3/1 -> ACC_P2_Targe/20(ObjectID)
  Selector2/1 -> ACC_P2_Targe/13(Object_VY)
  Selector5/1 -> ACC_P2_Targe/12(Object_VX)
  Selector6/1 -> ACC_P2_Targe/11(PP_ObjFusType_FC_Confirm)
  Selector7/1 -> ACC_P2_Targe/10(PP_ObjFusType_FR_Confirm)
  Selector8/1 -> ACC_P2_Targe/9(PP_ObjFusType_FC_FR_Confirm)
  Selector9/1 -> ACC_P2_Targe/8(Object_DY)
  Selector10/1 -> ACC_P2_Targe/7(Object_ObstacleProb)
  Selector11/1 -> ACC_P2_Targe/6(Object_Type)
  Selector15/1 -> ACC_P2_Targe/5(Object_DX)
  Selector16/1 -> ACC_P2_Targe/4(Object_HeadingAngle)
  Selector12/1 -> ACC_P2_Targe/3(PP_ObjMovingDirSignalProcessing)
  Selector13/1 -> ACC_P2_Targe/2(object_MovingState)
  Selector1/1 -> ACC_P2_Targe/1(Object_Fus_Type)
  ObjectID/1 -> Selector3/1
  ACC_Target_MovState_K2/1 -> ACC_P2_Targe/19(ACC_Target_MovState_K2)
  ACC_Target_MovState_K1/1 -> ACC_P2_Targe/18(ACC_Target_MovState_K1)
  ACC_Target_ID_K2/1 -> ACC_P2_Targe/17(ACC_Target_ID_K2)
  ACC_Target_ID_K1/1 -> ACC_P2_Targe/16(ACC_Target_ID_K1)
  SteerWheelAng/1 -> ACC_P2_Targe/15(SteerWheelAng)
  VIE_EgoVelocity/1 -> ACC_P2_Targe/14(VIE_EgoVelocity)
  Object_VY/1 -> Selector2/1
  Object_VX/1 -> Selector5/1
  PP_ObjFusType_FC_Confirm/1 -> Selector6/1
  PP_ObjFusType_FR_Confirm/1 -> Selector7/1
  PP_ObjFusType_FC_FR_Confirm/1 -> Selector8/1
  Object_DY/1 -> Selector9/1
  Object_ObstacleProb/1 -> Selector10/1
  Object_Type/1 -> Selector11/1
  Object_DX/1 -> Selector15/1
  Object_HeadingAngle/1 -> Selector16/1
  PP_ObjMovingDirSignalProcessing/1 -> Selector12/1
  object_MovingState/1 -> Selector13/1
  Object_Fus_Type/1 -> Selector1/1

== system PubIfDecisionTOS_MDL/TOS_20201112/TOS_2012080320/TOS/ACC/TOS_ACCLeftLane/ACC_LeftLane_Target/TOS_ACC_P2/ACC_P2_TargeDefault ==
  Action Port : ActionPort  ActionPortLabel=if(u1 ~= 0)
  Constant{1..6,8..13} (12 alike) : Constant  Value=0  OutDataTypeStr=boolean
  ACC_P2_TargeConfirm : Outport
  TOS_ACC_FusionType_ObserVale : Outport  Port=2
  TOS_ACC_TrgMovDir_ObserVale : Outport  Port=3
  TOS_ACC_TargetDxConfirm_ObserVale : Outport  Port=4
  TOS_ACC_ObjType_ObserVale : Outport  Port=5
  TOS_ACC_ObstacleProb_ObserVale : Outport  Port=6
  TOS_ACC_TrgMovDirFlag_1_ObserVale : Outport  Port=7
  TOS_ACC_TrgMovDirFlag_2_ObserVale : Outport  Port=8
  TOS_ACC_TrgMovDirFlag_3_ObserVale : Outport  Port=9
  TOS_ACC_TrgMovDirFlag_4_ObserVale : Outport  Port=10
  TOS_ACC_TrgMovDirFlag_5_ObserVale : Outport  Port=11
  TOS_ACC_TrgMovDirFlag_6_ObserVale : Outport  Port=12
  wires:
  Constant13/1 -> TOS_ACC_TrgMovDirFlag_6_ObserVale/1
  Constant12/1 -> TOS_ACC_TrgMovDirFlag_5_ObserVale/1
  Constant11/1 -> TOS_ACC_TrgMovDirFlag_4_ObserVale/1
  Constant10/1 -> TOS_ACC_TrgMovDirFlag_3_ObserVale/1
  Constant9/1 -> TOS_ACC_TrgMovDirFlag_2_ObserVale/1
  Constant8/1 -> TOS_ACC_TrgMovDirFlag_1_ObserVale/1
  Constant6/1 -> TOS_ACC_ObstacleProb_ObserVale/1
  Constant5/1 -> TOS_ACC_ObjType_ObserVale/1
  Constant4/1 -> TOS_ACC_TargetDxConfirm_ObserVale/1
  Constant3/1 -> TOS_ACC_TrgMovDir_ObserVale/1
  Constant1/1 -> TOS_ACC_FusionType_ObserVale/1
  Constant2/1 -> ACC_P2_TargeConfirm/1

== system PubIfDecisionTOS_MDL/TOS_20201112/TOS_2012080320/TOS/ACC/TOS_ACCLeftLane/ACC_LeftLane_Target/TOS_ACC_P4/ACC_P4_Targe ==
  ACC_P4_Index : Inport
  Object_Fus_Type : Inport  Port=2
  object_MovingState : Inport  Port=3
  PP_ObjMovingDirSignalProcessing : Inport  Port=4
  Object_HeadingAngle : Inport  Port=5
  Object_DX : Inport  Port=6
  Object_Type : Inport  Port=7
  Object_ObstacleProb : Inport  Port=8
  Object_DY : Inport  Port=9
  PP_ObjFusType_FC_FR_Confirm : Inport  Port=10
  PP_ObjFusType_FR_Confirm : Inport  Port=11
  PP_ObjFusType_FC_Confirm : Inport  Port=12
  Object_VX : Inport  Port=13
  Object_VY : Inport  Port=14
  VIE_EgoVelocity : Inport  Port=15
  SteerWheelAng : Inport  Port=16
  ACC_Target_ID_K1 : Inport  Port=17
  ACC_Target_ID_K2 : Inport  Port=18
  ACC_Target_MovState_K1 : Inport  Port=19
  ACC_Target_MovState_K2 : Inport  Port=20
  ObjectID : Inport  Port=21
  Action Port : ActionPort  ActionPortLabel=else
  ACC_P4_Targe : Subsystem
  Selector{1..3,5..13,15..16} (14 alike) : Selector  InputPortWidth=80  IndexOptions=Index vector (port)  Indices=[1 3]  OutputSizes=1
  ACC_P4_TargeConfirm : Outport
  TOS_ACC_FusionType_ObserVale : Outport  Port=2
  TOS_ACC_TrgMovDir_ObserVale : Outport  Port=3
  TOS_ACC_TargetDxConfirm_ObserVale : Outport  Port=4
  TOS_ACC_ObjType_ObserVale : Outport  Port=5
  TOS_ACC_ObstacleProb_ObserVale : Outport  Port=6
  TOS_ACC_TrgMovDirFlag_1_ObserVale : Outport  Port=7
  TOS_ACC_TrgMovDirFlag_2_ObserVale : Outport  Port=8
  TOS_ACC_TrgMovDirFlag_3_ObserVale : Outport  Port=9
  TOS_ACC_TrgMovDirFlag_4_ObserVale : Outport  Port=10
  TOS_ACC_TrgMovDirFlag_5_ObserVale : Outport  Port=11
  TOS_ACC_TrgMovDirFlag_6_ObserVale : Outport  Port=12
  wires:
  Object_Fus_Type/1 -> Selector1/1
  object_MovingState/1 -> Selector13/1
  PP_ObjMovingDirSignalProcessing/1 -> Selector12/1
  Object_HeadingAngle/1 -> Selector16/1
  Object_DX/1 -> Selector15/1
  Object_Type/1 -> Selector11/1
  Object_ObstacleProb/1 -> Selector10/1
  Object_DY/1 -> Selector9/1
  PP_ObjFusType_FC_FR_Confirm/1 -> Selector8/1
  PP_ObjFusType_FR_Confirm/1 -> Selector7/1
  PP_ObjFusType_FC_Confirm/1 -> Selector6/1
  Object_VX/1 -> Selector5/1
  Object_VY/1 -> Selector2/1
  VIE_EgoVelocity/1 -> ACC_P4_Targe/14(VIE_EgoVelocity)
  SteerWheelAng/1 -> ACC_P4_Targe/15(SteerWheelAng)
  ACC_Target_ID_K1/1 -> ACC_P4_Targe/16(ACC_Target_ID_K1)
  ACC_Target_ID_K2/1 -> ACC_P4_Targe/17(ACC_Target_ID_K2)
  ACC_Target_MovState_K1/1 -> ACC_P4_Targe/18(ACC_Target_MovState_K1)
  ACC_Target_MovState_K2/1 -> ACC_P4_Targe/19(ACC_Target_MovState_K2)
  ObjectID/1 -> Selector3/1
  Selector1/1 -> ACC_P4_Targe/1(Object_Fus_Type)
  Selector13/1 -> ACC_P4_Targe/2(object_MovingState)
  Selector12/1 -> ACC_P4_Targe/3(PP_ObjMovingDirSignalProcessing)
  Selector16/1 -> ACC_P4_Targe/4(Object_HeadingAngle)
  Selector15/1 -> ACC_P4_Targe/5(Object_DX)
  Selector11/1 -> ACC_P4_Targe/6(Object_Type)
  Selector10/1 -> ACC_P4_Targe/7(Object_ObstacleProb)
  Selector9/1 -> ACC_P4_Targe/8(Object_DY)
  Selector8/1 -> ACC_P4_Targe/9(PP_ObjFusType_FC_FR_Confirm)
  Selector7/1 -> ACC_P4_Targe/10(PP_ObjFusType_FR_Confirm)
  Selector6/1 -> ACC_P4_Targe/11(PP_ObjFusType_FC_Confirm)
  Selector5/1 -> ACC_P4_Targe/12(Object_VX)
  Selector2/1 -> ACC_P4_Targe/13(Object_VY)
  Selector3/1 -> ACC_P4_Targe/20(ObjectID)
  ACC_P4_Index/1 -> Selector1/2, Selector13/2, Selector12/2, Selector15/2, Selector11/2, Selector10/2, Selector9/2, Selector8/2, Selector7/2, Selector6/2, Selector5/2, Selector2/2, Selector3/2, Selector16/2
  ACC_P4_Targe/6(TOS_ACC_ObstacleProb_ObserVale) -> TOS_ACC_ObstacleProb_ObserVale/1
  ACC_P4_Targe/5(TOS_ACC_ObjType_ObserVale) -> TOS_ACC_ObjType_ObserVale/1
  ACC_P4_Targe/7(TOS_ACC_TrgMovDirFlag_1_ObserVale) -> TOS_ACC_TrgMovDirFlag_1_ObserVale/1
  ACC_P4_Targe/4(TOS_ACC_TargetDxConfirm_ObserVale) -> TOS_ACC_TargetDxConfirm_ObserVale/1
  ACC_P4_Targe/8(TOS_ACC_TrgMovDirFlag_2_ObserVale) -> TOS_ACC_TrgMovDirFlag_2_ObserVale/1
  ACC_P4_Targe/3(TOS_ACC_TrgMovDir_ObserVale) -> TOS_ACC_TrgMovDir_ObserVale/1
  ACC_P4_Targe/9(TOS_ACC_TrgMovDirFlag_3_ObserVale) -> TOS_ACC_TrgMovDirFlag_3_ObserVale/1
  ACC_P4_Targe/2(TOS_ACC_FusionType_ObserVale) -> TOS_ACC_FusionType_ObserVale/1
  ACC_P4_Targe/10(TOS_ACC_TrgMovDirFlag_4_ObserVale) -> TOS_ACC_TrgMovDirFlag_4_ObserVale/1
  ACC_P4_Targe/1(ACC_P4_TargeConfirm) -> ACC_P4_TargeConfirm/1
  ACC_P4_Targe/11(TOS_ACC_TrgMovDirFlag_5_ObserVale) -> TOS_ACC_TrgMovDirFlag_5_ObserVale/1
  ACC_P4_Targe/12(TOS_ACC_TrgMovDirFlag_6_ObserVale) -> TOS_ACC_TrgMovDirFlag_6_ObserVale/1

== system PubIfDecisionTOS_MDL/TOS_20201112/TOS_2012080320/TOS/ACC/TOS_ACCLeftLane/ACC_LeftLane_Target/TOS_ACC_P4/ACC_P4_TargeDefault ==
  Action Port : ActionPort  ActionPortLabel=if(u1 ~= 0)
  Constant{1..6,8..13} (12 alike) : Constant  Value=0  OutDataTypeStr=boolean
  ACC_P4_TargeConfirm : Outport
  TOS_ACC_FusionType_ObserVale : Outport  Port=2
  TOS_ACC_TrgMovDir_ObserVale : Outport  Port=3
  TOS_ACC_TargetDxConfirm_ObserVale : Outport  Port=4
  TOS_ACC_ObjType_ObserVale : Outport  Port=5
  TOS_ACC_ObstacleProb_ObserVale : Outport  Port=6
  TOS_ACC_TrgMovDirFlag_1_ObserVale : Outport  Port=7
  TOS_ACC_TrgMovDirFlag_2_ObserVale : Outport  Port=8
  TOS_ACC_TrgMovDirFlag_3_ObserVale : Outport  Port=9
  TOS_ACC_TrgMovDirFlag_4_ObserVale : Outport  Port=10
  TOS_ACC_TrgMovDirFlag_5_ObserVale : Outport  Port=11
  TOS_ACC_TrgMovDirFlag_6_ObserVale : Outport  Port=12
  wires:
  Constant2/1 -> ACC_P4_TargeConfirm/1
  Constant1/1 -> TOS_ACC_FusionType_ObserVale/1
  Constant3/1 -> TOS_ACC_TrgMovDir_ObserVale/1
  Constant4/1 -> TOS_ACC_TargetDxConfirm_ObserVale/1
  Constant5/1 -> TOS_ACC_ObjType_ObserVale/1
  Constant6/1 -> TOS_ACC_ObstacleProb_ObserVale/1
  Constant8/1 -> TOS_ACC_TrgMovDirFlag_1_ObserVale/1
  Constant9/1 -> TOS_ACC_TrgMovDirFlag_2_ObserVale/1
  Constant10/1 -> TOS_ACC_TrgMovDirFlag_3_ObserVale/1
  Constant11/1 -> TOS_ACC_TrgMovDirFlag_4_ObserVale/1
  Constant12/1 -> TOS_ACC_TrgMovDirFlag_5_ObserVale/1
  Constant13/1 -> TOS_ACC_TrgMovDirFlag_6_ObserVale/1

== system PubIfDecisionTOS_MDL/TOS_20201112/TOS_2012080320/TOS/ACC/TOS_ACCLeftLane/ACC_Object_PreConfirm/ACC_Object_PreConfirm/ACC_Object_PreConfirm ==
  Object_ID : Inport
  PP_ObjFusType_FC_FR_Confirm : Inport  Port=2
  PP_ObjFusType_FR_Confirm : Inport  Port=3
  PP_ObjFusType_FC_Confirm : Inport  Port=4
  Obj_MovingState : Inport  Port=5
  Obj_Dx : Inport  Port=6
  Object_ObstacleProb : Inport  Port=7
  Object_DY : Inport  Port=8
  Object_ObjType : Inport  Port=9
  ACC_Target_ID_K1 : Inport  Port=10
  ACC_Target_Dx_K1 : Inport  Port=11
  Action Port : ActionPort  ActionPortLabel=else
  " " : Subsystem
  Bus Creator : BusCreator  Inputs=11
  Bus Selector1 : BusSelector  OutputSignals=PP_ObjFusType_FC_Confirm,Obj_MovingState
  Bus Selector2 : BusSelector  OutputSignals=PP_ObjFusType_FC_FR_Confirm,PP_ObjFusType_FC_Confirm,PP_ObjFusType_FR_Confirm
  Bus Selector4 : BusSelector  OutputSignals=Object_ObjType
  Constant1 : Constant  OutDataTypeStr=boolean
  Logical Operator1 : Logic  Inputs=4  AllPortsSameDT=off  OutDataTypeStr=boolean
  Subsystem : Subsystem
  Subsystem1 : Subsystem
  TOS_ACC_DyConfirm : Subsystem
  Terminator : Terminator
  TOS_ACC_TargetPre_Confirm_FiltFlag : Outport
  TOS_ACC_TargetPre_FusionTypeFlag_ObserVale : Outport  Port=2
  TOS_ACC_TargetPre_PassedbyTarget_ObserVale : Outport  Port=3
  TOS_ACC_TargetPre_ObjType_ObserVale : Outport  Port=4
  TOS_ACC_DyConfirm_ObserVale : Outport  Port=5
  wires:
  Subsystem/1(TOS_ACC_TargetPre_TargetFusionTypeFlag) -> [TOS_ACC_TargetPre_FusionTypeFlag_ObserVale], Logical Operator1/1
  Subsystem1/1(TOS_ACC_TargetPre_ObjectPassedbyTarget_Flag) -> [TOS_ACC_TargetPre_PassedbyTarget_Flag_ObserVale], Logical Operator1/2
  PP_ObjFusType_FR_Confirm/1 -> Bus Creator/3  "PP_ObjFusType_FR_Confirm"
  Object_ID/1 -> Bus Creator/1  "Object_ID"
  PP_ObjFusType_FC_Confirm/1 -> Bus Creator/4  "PP_ObjFusType_FC_Confirm"
  Bus Selector2/1 -> Subsystem/1(PP_ObjFusType_FC_FR_Confirm)  "<PP_ObjFusType_FC_FR_Confirm>"
  Bus Selector2/3 -> Subsystem/3(PP_ObjFusType_FC_Confirm)  "<PP_ObjFusType_FR_Confirm>"
  Bus Selector1/1 -> Subsystem1/1(PP_ObjFusType_FC_Confirm)  "<PP_ObjFusType_FC_Confirm>"
  Bus Selector2/2 -> Subsystem/2(PP_ObjFusType_FR_Confirm)  "<PP_ObjFusType_FC_Confirm>"
  PP_ObjFusType_FC_FR_Confirm/1 -> Bus Creator/2  "PP_ObjFusType_FC_FR_Confirm"
  ACC_Target_ID_K1/1 -> Bus Creator/10  "ACC_Target_ID_K1"
  Object_DY/1 -> Bus Creator/8  "Object_DY"
  Bus Selector1/2 -> Subsystem1/2(Obj_MovingState)  "<Obj_MovingState>"
  ACC_Target_Dx_K1/1 -> Bus Creator/11  "ACC_Target_Dx_K1"
  Obj_MovingState/1 -> Bus Creator/5  "Obj_MovingState"
  Object_ObstacleProb/1 -> Bus Creator/7  "Object_ObstacleProb"
  Obj_Dx/1 -> Bus Creator/6  "Obj_Dx"
  Bus Selector4/1 -> " "/1(Object_Type)  "<Object_ObjType>"
  " "/1(TOS_ACC_TargetPre_ObjType) -> Logical Operator1/3, [TOS_ACC_TargetPre_ObjType_ObserVale]
  Object_ObjType/1 -> Bus Creator/9  "Object_ObjType"
  [TOS_ACC_TargetPre_FusionTypeFlag_ObserVale] -> TOS_ACC_TargetPre_FusionTypeFlag_ObserVale/1
  [TOS_ACC_TargetPre_PassedbyTarget_Flag_ObserVale] -> TOS_ACC_TargetPre_PassedbyTarget_ObserVale/1
  [TOS_ACC_TargetPre_ObjType_ObserVale] -> TOS_ACC_TargetPre_ObjType_ObserVale/1
  Constant1/1 -> Logical Operator1/4, [TOS_ACC_DyConfirm_ObserVale]
  [TOS_ACC_DyConfirm_ObserVale] -> TOS_ACC_DyConfirm_ObserVale/1
  Logical Operator1/1 -> TOS_ACC_TargetPre_Confirm_FiltFlag/1
  Bus Creator/1 -> TOS_ACC_DyConfirm/1(TOS_ACC_Dy), Bus Selector4/1, Bus Selector1/1, Bus Selector2/1
  TOS_ACC_DyConfirm/1(TOS_ACC_TargetPre_DyConfirm) -> Terminator/1

== system PubIfDecisionTOS_MDL/TOS_20201112/TOS_2012080320/TOS/ACC/TOS_ACCLeftLane/ACC_Object_PreConfirm/ACC_Object_PreConfirm/ACC_Object_PreConfirmDefault ==
  Action Port : ActionPort  ActionPortLabel=if(u1 ~= 0)
  Constant{2,5..6,8,10} (5 alike) : Constant  Value=0  OutDataTypeStr=boolean
  TOS_ACC_TargetPre_Confirm_FiltFlag : Outport
  TOS_ACC_TargetPre_FusionTypeFlag_ObserVale : Outport  Port=2
  TOS_ACC_TargetPre_PassedbyTarget_ObserVale : Outport  Port=3
  TOS_ACC_TargetPre_ObjType_ObserVale : Outport  Port=4
  TOS_ACC_DyConfirm_ObserVale : Outport  Port=5
  wires:
  Constant2/1 -> TOS_ACC_TargetPre_Confirm_FiltFlag/1
  Constant5/1 -> TOS_ACC_TargetPre_FusionTypeFlag_ObserVale/1
  Constant6/1 -> TOS_ACC_TargetPre_PassedbyTarget_ObserVale/1
  Constant8/1 -> TOS_ACC_TargetPre_ObjType_ObserVale/1
  Constant10/1 -> TOS_ACC_DyConfirm_ObserVale/1
